simulink model "S_Med_TE_MPPT_Simp_V1"  (R2017a)
settings: Solver=FixedStepDiscrete  StartTime=0.0  StopTime=10.0  RelTol=1e-3
values from neighbouring files (symbols this model uses):
  A = [0 (d-1)/L ... (first row only)    [M_Mod_Sim_PV_V1.m]
  dIL = (vpv/L)*d*Ts1    (= 0.460350492963)    [M_Mod_Sim_PV_V1.m]
  Kf1 = Scala/dDmax    (= 5.88235294118)    [M_Mod_Sim_PV_V1.m]
  ki = 1/ipv    (= 0.0636345580933)    [M_Mod_Sim_PV_V1.m]
  Ts_Ma = 10e-3    (= 0.01)    [M_Mod_Sim_PV_V1.m]
undefined symbols (not defined in the file or in its folder): Down, GPTRIP1SEL, GPTRIP2SEL, TZ1, TZ2, Up
libraries: c2802xlib x4, c2806xlib x2, fuzblock x1
settings Model: ExtModeTrigDuration=8  Creator=dricl  LastModifiedBy=dricl
settings OptimizationCC: DefaultUnderspecifiedDataType=single  PassReuseOutputArgsAs=Individual arguments  MaxStackSize=512
settings DebuggingCC: ParameterTunabilityLossMsg=error
settings HardwareCC: ProdBitPerChar=16  ProdBitPerInt=16  ProdBitPerPointer=32  ProdBitPerSizeT=32  ProdBitPerPtrDiffT=32  ProdLargestAtomicInteger=Integer  ProdLargestAtomicFloat=None  ProdWordSize=16  ProdLongLongMode=on  ProdHWDeviceType=Texas Instruments->C2000
settings SFSimCC: MATLABDynamicMemAlloc=off
settings RTWCC: SystemTargetFile=ert.tlc  HardwareBoard=TI Piccolo F2806x  TLCOptions=-aInlineSetEventsForThisBaseRateFcn=TLC_FALSE -aSuppressMultiTaskScheduler=TLC_FALSE -aRateBasedStepFcn=1  TemplateMakefile=ert_default_tmf  Description=Embedded Coder  Toolchain=Texas Instruments Code Composer Studio v5 (C2000)  CodeExecutionProfiling=on  CodeProfilingSaveOptions=AllData  CodeProfilingInstrumentation=on
settings CodeAppCC: ForceParamTrailComments=on  IgnoreCustomStorageClasses=off  OperatorAnnotations=on  SimulinkDataObjDesc=on  SFDataObjDesc=on  MATLABFcnDesc=on  InsertBlockDesc=on  MATLABSourceComments=on
settings ERTTargetCC: CodeReplacementLibrary=TI C28x  MemSecPackage=tic2000demospkg  MemSecFuncExecute=code_ramfuncs

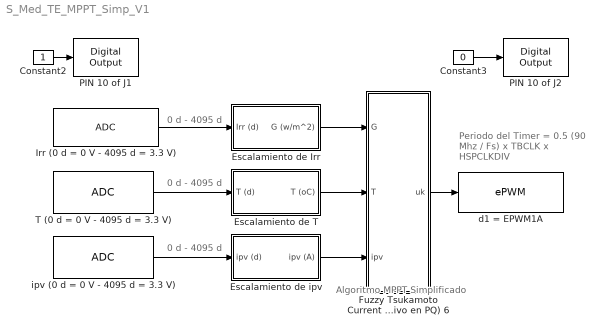
== system S_Med_TE_MPPT_Simp_V1 ==
  note: 0 d - 4095 d
  note: Periodo del Timer =
      |  0.5 (90 Mhz / Fs)  x
      | TBCLK x HSPCLKDIV
  note: 0 d - 4095 d
  note: 0 d - 4095 d
  note: Algoritmo MPPT Simplificado
  Constant2 : Constant  Priority=1  SampleTime=Ts_Ma
  Constant3 : Constant  Priority=11  Value=0  SampleTime=Ts_Ma
  Escalamiento de Irr : Subsystem  Priority=6  TreatAsAtomicUnit=on
  Escalamiento de T : Subsystem  Priority=7  TreatAsAtomicUnit=on
  Escalamiento de ipv : Subsystem  Priority=8  TreatAsAtomicUnit=on
  "Fuzzy Tsukamoto Current Controller n_mppt = 99.11%, ta(2%) = 0.12 s con Steps de Irrad Interv. 2 Seg. n_mppt = 96.74%, ta(2%) = 0.12 s con Steps de Irrad Interv. 0.5 Seg. n_mppt = 99.37%, ta(2%) = 0.12 s con Curva de Irrad Este controlador puede disminuir ta e incrementar a tr para mitigar los MP en id (impacto positivo en PQ) 6" : Subsystem  Priority=9
  "Irr (0 d = 0 V - 4095 d = 3.3 V) " : c2802xlib/ADC  Priority=3  ADCModule=1  samplingMode=Single sample mode  ADCResolution=12-bit (Single-ended input)  useSOC1=SOC1  useSOC2=SOC0_SOC1  SOCAcquisitionWindow=7  SOCTriggerSource=ePWM1_ADCSOCA  SOCInterruptTrigger=No ADCINT  Ts=Ts_Ma  dType=uint16  postInterrupt=off  interruptSel=ADCINT1  ADCINTContinuous=on  endma=off  chdma=1  blkParamProc=C2000  conv1=ADCINA1  conv2=ADCINA0 and ADCINB0  conv1_Type4=ADCIN0  conv2_Type4=ADCIN0 and ADCIN1
      settings: SourceProductName=Embedded Coder Support Package for Texas Instruments C2000 Processors
  PIN 10 of J1 : c2806xlib/Digital Output  Priority=2  GPIO_Number=GPIO32~GPIO39  GPIO_Bit0=on  GPIO_BIT0_Toggle=off  GPIO_Bit1=off  GPIO_BIT1_Toggle=off  GPIO_Bit2=off  GPIO_BIT2_Toggle=off  GPIO_Bit3=off  GPIO_BIT3_Toggle=off  GPIO_Bit4=off  GPIO_BIT4_Toggle=off  GPIO_Bit5=off  GPIO_BIT5_Toggle=off  GPIO_Bit6=off  GPIO_BIT6_Toggle=off  GPIO_Bit7=off  GPIO_BIT7_Toggle=off
      settings: SourceProductName=Embedded Coder Support Package for Texas Instruments C2000 Processors  SourceProductBaseCode=TIC2000
  PIN 10 of J2 : c2806xlib/Digital Output  Priority=12  GPIO_Number=GPIO32~GPIO39  GPIO_Bit0=on  GPIO_BIT0_Toggle=off  GPIO_Bit1=off  GPIO_BIT1_Toggle=off  GPIO_Bit2=off  GPIO_BIT2_Toggle=off  GPIO_Bit3=off  GPIO_BIT3_Toggle=off  GPIO_Bit4=off  GPIO_BIT4_Toggle=off  GPIO_Bit5=off  GPIO_BIT5_Toggle=off  GPIO_Bit6=off  GPIO_BIT6_Toggle=off  GPIO_Bit7=off  GPIO_BIT7_Toggle=off
      settings: SourceProductName=Embedded Coder Support Package for Texas Instruments C2000 Processors  SourceProductBaseCode=TIC2000
  "T (0 d = 0 V - 4095 d = 3.3 V) " : c2802xlib/ADC  Priority=4  ADCModule=1  samplingMode=Single sample mode  ADCResolution=12-bit (Single-ended input)  useSOC1=SOC3  useSOC2=SOC0_SOC1  SOCAcquisitionWindow=7  SOCTriggerSource=ePWM1_ADCSOCA  SOCInterruptTrigger=No ADCINT  Ts=Ts_Ma  dType=uint16  postInterrupt=off  interruptSel=ADCINT1  ADCINTContinuous=on  endma=off  chdma=1  blkParamProc=C2000  conv1=ADCINA2  conv2=ADCINA0 and ADCINB0  conv1_Type4=ADCIN0  conv2_Type4=ADCIN0 and ADCIN1
      settings: SourceProductName=Embedded Coder Support Package for Texas Instruments C2000 Processors
  d1 = EPWM1A : c2802xlib/ePWM  Priority=10  useModule=ePWM1  ePWMxLINKTBPRD=Not Linked  periodUnits=Clock cycles  timerSource=Specify via dialog  timerPeriod_clk=9000  timerPeriod_sec=0.0001  tbshadow=Counter equals to zero  countingMode=Up-Down  phaseActiveEnable=Disable  phaseDirection=Count down after sync  phaseActive=0  synchronizationEnable=off  dcaevt1Sync=off  dcbevt1Sync=off  synchronizationOption=Disable  clockPrescale=1  HSclockPrescale=1  enswap=off  ePWMxAStatus=on  ePWMxAactionLogic1=Do nothing  ePWMxAactionLogic2=Do nothing  ePWMxAactionLogic3=Clear  ePWMxAactionLogic4=Set  ePWMxAactionLogic5=Do nothing  ePWMxAactionLogic6=Do nothing  ePWMxALoadMode=Load on counter equals to zero (CTR=Zero)  ePWMxACSFenable=off  ePWMxACSFvalue=Forcing disable  ePWMxASFreload=Zero  ePWMxBStatus=off  ePWMxBactionLogic1=Set  ePWMxBactionLogic2=Clear  ePWMxBactionLogic3=Do nothing  ePWMxBactionLogic4=Do nothing  ePWMxBactionLogic5=Clear  ePWMxBactionLogic6=Set  ePWMxBLoadMode=Load on counter equals to zero (CTR=Zero)  ePWMxBCSFenable=off  ePWMxBCSFvalue=Forcing disable  ePWMxBSFreload=Zero  ePWNxBOutWay=off  ePWMxLINKCMPA=Not Linked  CMPAUnits=Clock cycles  CMPASource=Input port  CMPAValue_per=50  CMPAValue_clk=4500  enCMPAshadow=Counter equals to zero  ePWMxLINKCMPB=Not Linked  CMPBUnits=Clock cycles  CMPBSource=Specify via dialog  CMPBValue_per=50  CMPBValue_clk=4500  enCMPBshadow=Counter equals to zero  ePWMxLINKCMPC=Not Linked  CMPCUnits=Clock cycles  CMPCSource=Specify via dialog  CMPCValue_per=50  CMPCValue_clk=32000  enCMPCshadow=Counter equals to zero  ePWMxLINKCMPD=Not Linked  CMPDUnits=Clock cycles  CMPDSource=Specify via dialog  CMPDValue_per=50  CMPDValue_clk=32000  enCMPDshadow=Counter equals to zero  enableDBePWMxA=on  enableDBePWMxB=on  enhalfcycle=off  DBpolarity=Active high complementary (AHC)  DBedgeDelay=Positive  DBSource_ePWMxA=ePWMxA  DBSource_ePWMxB=ePWMxA  DBperiodSource=Specify via dialog  REDperiod=50  FEDperiod=50  adcstartModuleA=on  adcrequestEventA=First event  adcstartEventA=Counter equals to period (CTR=PRD)  adcstartEventA_type2=Digital Compare Module A Event 1 start of conversion (DCAEVT1.soc)  adcstartModuleB=off  adcrequestEventB=First event  adcstartEventB=Counter equals to zero (CTR=Zero)  adcstartEventB_type2=Counter equals to zero (CTR=Zero)  intEn=off  intPrd=First event  intSel=Counter equals to zero (CTR=Zero)  intSel_type2=Counter equals to zero (CTR=Zero)  hrpe=off  enHRPWM=off  HRPWM_LoadMode=Counter equals to period (CTR=PRD)  HRPWM_CTLMode=Duty or Period control mode  HRPWM_EDGMode=Both edge  hrpeb=off  enHRPWMB=off  HRPWM_LoadModeB=Counter equals to zero (CTR=ZERO)  HRPWM_CTLModeB=Duty or Period control mode  HRPWM_EDGModeB=Both edge  enSFO=on  enautoconv=on  chopperEnable=off  chopperFrequency=1  chopperFirstwidth=1  chopperDuty=12.5%  tripZonesource=Specify via dialog  tzselOSHT1=off  tzselOSHT2=off  tzselOSHT3=off  tzselOSHDCAEV1=off  tzselOSHDCBEV1=off  tzselCBC1=off  tzselCBC2=off  tzselCBC3=off  tzselCBCDCAEV2=off  tzselCBCDCBEV2=off  tzselOSHT4=off  tzselOSHT5=off  tzselOSHT6=off  tzselCBC4=off  tzselCBC5=off  tzselCBC6=off  enTzOstIntr=off  enTzCbcIntr=off  enTzDCAEVT1Intr=off  enTzDCAEVT2Intr=off  enTzDCBEVT1Intr=off  enTzDCBEVT2Intr=off  ePWMxAforced=No action  ePWMxBforced=No action  DCAEVT1forced=No action  DCBEVT1forced=No action  DCAEVT2forced=No action  DCBEVT2forced=No action  dcah=Trip Zone 1 input (TZ1)  dcal=Trip Zone 2 input (TZ2)  dcbh=Trip Zone 1 input (TZ1)  dcbl=Trip Zone 2 input (TZ2)  dcah_type2=GPTRIP1SEL/(TZ1)  dcal_type2=GPTRIP2SEL/(TZ2)  dcbh_type2=GPTRIP1SEL/(TZ1)  dcbl_type2=GPTRIP2SEL/(TZ2)  gendcaevt1=Event disabled  gendcaevt2=Event disabled  gendcbevt1=Event disabled  gendcbevt2=Event disabled  dcaevt1src=DCAEVT1 with sync  dcaevt2src=DCAEVT2 with sync  dcbevt1src=DCBEVT1 with sync  dcbevt2src=DCBEVT2 with sync  pulsesel=Counter equals to zero (CTR=Zero)  blankinv=off  blankoffset=0  blankwidth=0  evsrcsel=Filtered version of DCAEVT1 (DCAEVT1FILT)  encape=off  PwmType=C2000
      settings: SourceProductName=Embedded Coder Support Package for Texas Instruments C2000 Processors
  "ipv (0 d = 0 V - 4095 d = 3.3 V) " : c2802xlib/ADC  Priority=5  ADCModule=1  samplingMode=Single sample mode  ADCResolution=12-bit (Single-ended input)  useSOC1=SOC2  useSOC2=SOC0_SOC1  SOCAcquisitionWindow=7  SOCTriggerSource=ePWM1_ADCSOCA  SOCInterruptTrigger=No ADCINT  Ts=Ts_Ma  dType=uint16  postInterrupt=off  interruptSel=ADCINT1  ADCINTContinuous=on  endma=off  chdma=1  blkParamProc=C2000  conv1=ADCINA0  conv2=ADCINA0 and ADCINB0  conv1_Type4=ADCIN0  conv2_Type4=ADCIN0 and ADCIN1
      settings: SourceProductName=Embedded Coder Support Package for Texas Instruments C2000 Processors
  wires:
  "ipv (0 d = 0 V - 4095 d = 3.3 V) "/1 -> Escalamiento de ipv/1(ipv (d))
  "Irr (0 d = 0 V - 4095 d = 3.3 V) "/1 -> Escalamiento de Irr/1(Irr (d))
  Constant2/1 -> PIN 10 of J1/1
  Constant3/1 -> PIN 10 of J2/1
  "T (0 d = 0 V - 4095 d = 3.3 V) "/1 -> Escalamiento de T/1(T (d))
  Escalamiento de Irr/1(G (w/m^2)) -> "Fuzzy Tsukamoto Current Controller n_mppt = 99.11%, ta(2%) = 0.12 s con Steps de Irrad Interv. 2 Seg. n_mppt = 96.74%, ta(2%) = 0.12 s con Steps de Irrad Interv. 0.5 Seg. n_mppt = 99.37%, ta(2%) = 0.12 s con Curva de Irrad Este controlador puede disminuir ta e incrementar a tr para mitigar los MP en id (impacto positivo en PQ) 6"/1(G)
  Escalamiento de T/1(T (oC)) -> "Fuzzy Tsukamoto Current Controller n_mppt = 99.11%, ta(2%) = 0.12 s con Steps de Irrad Interv. 2 Seg. n_mppt = 96.74%, ta(2%) = 0.12 s con Steps de Irrad Interv. 0.5 Seg. n_mppt = 99.37%, ta(2%) = 0.12 s con Curva de Irrad Este controlador puede disminuir ta e incrementar a tr para mitigar los MP en id (impacto positivo en PQ) 6"/2(T)
  Escalamiento de ipv/1(ipv (A)) -> "Fuzzy Tsukamoto Current Controller n_mppt = 99.11%, ta(2%) = 0.12 s con Steps de Irrad Interv. 2 Seg. n_mppt = 96.74%, ta(2%) = 0.12 s con Steps de Irrad Interv. 0.5 Seg. n_mppt = 99.37%, ta(2%) = 0.12 s con Curva de Irrad Este controlador puede disminuir ta e incrementar a tr para mitigar los MP en id (impacto positivo en PQ) 6"/3(ipv)
  "Fuzzy Tsukamoto Current Controller n_mppt = 99.11%, ta(2%) = 0.12 s con Steps de Irrad Interv. 2 Seg. n_mppt = 96.74%, ta(2%) = 0.12 s con Steps de Irrad Interv. 0.5 Seg. n_mppt = 99.37%, ta(2%) = 0.12 s con Curva de Irrad Este controlador puede disminuir ta e incrementar a tr para mitigar los MP en id (impacto positivo en PQ) 6"/1(uk) -> d1 = EPWM1A/1

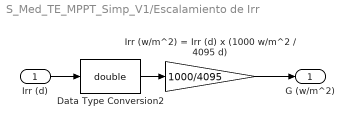
== system S_Med_TE_MPPT_Simp_V1/Escalamiento de Irr ==
  Irr (d) : Inport
  Data Type Conversion2 : DataTypeConversion  OutDataTypeStr=double
  Irr (w/m^2) = Irr (d) x (1000 w/m^2 / 4095 d) : Gain  Gain=1000/4095
  G (w/m^2) : Outport
  wires:
  Irr (d)/1 -> Data Type Conversion2/1
  Data Type Conversion2/1 -> Irr (w/m^2) = Irr (d) x (1000 w/m^2 / 4095 d)/1
  Irr (w/m^2) = Irr (d) x (1000 w/m^2 / 4095 d)/1 -> G (w/m^2)/1

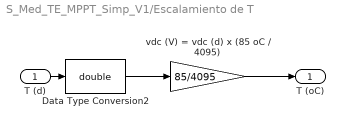
== system S_Med_TE_MPPT_Simp_V1/Escalamiento de T ==
  T (d) : Inport
  Data Type Conversion2 : DataTypeConversion  OutDataTypeStr=double
  vdc (V) = vdc (d) x (85 oC / 4095) : Gain  Gain=85/4095
  T (oC) : Outport
  wires:
  Data Type Conversion2/1 -> vdc (V) = vdc (d) x (85 oC / 4095)/1
  T (d)/1 -> Data Type Conversion2/1
  vdc (V) = vdc (d) x (85 oC / 4095)/1 -> T (oC)/1

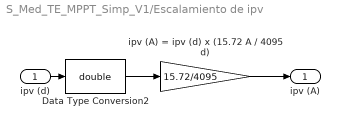
== system S_Med_TE_MPPT_Simp_V1/Escalamiento de ipv ==
  ipv (d) : Inport
  Data Type Conversion2 : DataTypeConversion  OutDataTypeStr=double
  ipv (A) = ipv (d) x (15.72 A / 4095 d) : Gain  Gain=15.72/4095
  ipv (A) : Outport
  wires:
  ipv (d)/1 -> Data Type Conversion2/1
  Data Type Conversion2/1 -> ipv (A) = ipv (d) x (15.72 A / 4095 d)/1
  ipv (A) = ipv (d) x (15.72 A / 4095 d)/1 -> ipv (A)/1

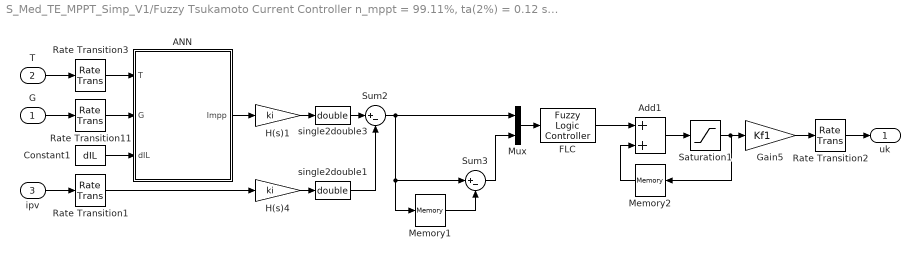
== system S_Med_TE_MPPT_Simp_V1/Fuzzy Tsukamoto Current Controller n_mppt = 99.11%, ta(2%) = 0.12 s con Steps de Irrad Interv. 2 Seg. n_mppt = 96.74%, ta(2%) = 0.12 s con Steps de Irrad Interv. 0.5 Seg. n_mppt = 99.37%, ta(2%) = 0.12 s con Curva de Irrad Este controlador puede disminuir ta e incrementar a tr para mitigar los MP en id (impacto positivo en PQ) 6 ==
  G : Inport
  T : Inport  Port=2
  ipv : Inport  Port=3
  ANN : MATLAB Function  TreatAsAtomicUnit=on
  Add1 : Sum
  Constant1 : Constant  Value=dIL  SampleTime=Ts_Ma
  FLC : fuzblock/Fuzzy Logic  Controller  fis=['5_Rules_MaMPPTCtrl_V1.fis']
  Gain5 : Gain  Gain=Kf1
  H(s)1 : Gain  Gain=ki
  H(s)4 : Gain  Gain=ki
  Memory1 : Memory  InheritSampleTime=on
  Memory2 : Memory  InheritSampleTime=on
  Mux : Mux  Inputs=2
  Rate Transition{1..3,11} (4 alike) : RateTransition  Deterministic=off  OutPortSampleTime=Ts_Ma
  Saturation1 : Saturate  UpperLimit=1  LowerLimit=0
  Sum2 : Sum  Inputs=|+-
  Sum3 : Sum  Inputs=|+-
  single2double1 : DataTypeConversion  OutDataTypeStr=double
  single2double3 : DataTypeConversion  OutDataTypeStr=double
  uk : Outport
  wires:
  Rate Transition2/1 -> uk/1
  Memory2/1 -> Add1/2
  single2double3/1 -> Sum2/1
  single2double1/1 -> Sum2/2
  Rate Transition1/1 -> H(s)4/1
  ipv/1 -> Rate Transition1/1
  Memory1/1 -> Sum3/2
  Add1/1 -> Saturation1/1
  Saturation1/1 -> Memory2/1, Gain5/1
  Gain5/1 -> Rate Transition2/1
  H(s)1/1 -> single2double3/1
  H(s)4/1 -> single2double1/1
  Mux/1 -> FLC/1
  Sum2/1 -> Memory1/1, Sum3/1, Mux/1
  Sum3/1 -> Mux/2
  FLC/1 -> Add1/1
  Rate Transition11/1 -> ANN/2(G)
  Rate Transition3/1 -> ANN/1(T)
  G/1 -> Rate Transition11/1
  T/1 -> Rate Transition3/1
  Constant1/1 -> ANN/3(dIL)
  ANN/1(Impp) -> H(s)1/1

== matlab function S_Med_TE_MPPT_Simp_V1/Fuzzy Tsukamoto Current Controller n_mppt = 99.11%, ta(2%) = 0.12 s con Steps de Irrad Interv. 2 Seg. n_mppt = 96.74%, ta(2%) = 0.12 s con Steps de Irrad Interv. 0.5 Seg. n_mppt = 99.37%, ta(2%) = 0.12 s con Curva de Irrad Este controlador puede disminuir ta e incrementar a tr para mitigar los MP en id (impacto positivo en PQ) 6/ANN ==
  data: T input; G input; Impp output; dIL input
function Impp = ANN(T,G,dIL)

persistent w1 w2 b1 b2
persistent Media_T Media_G Media_Impp
persistent Std_T Std_G Std_Impp

if isempty(w1)

    w1 = [ ...
    0.0800025921861489, -0.2701751801560736; ...
    0.0593520039763442, -0.2027427120547354; ...
    0.5243220553759315, 0.1630350434999212; ...
    1.5863696961889453, 0.1819964305283979; ...
    -6.2441844424671862, -2.3703350404983592];

    w2 = [-8.8999407900435337, -14.3986509522404820, 2.0426767954493643, 0.2264966677997083, -0.0152565567604669];

    b1 = [-1.5663442358887940, 0.9898870290888165, -0.3688041794616991, 2.4837588514086595, -13.7136306663382130];

    b2 = 10.9993641444783350;

    Media_T = 30.0000000000000000;
    Media_G = 650.0000000000000000;
    Media_Impp = 10.2067479487858090;

    Std_T = 32.3328756401525790;
    Std_G = 324.7437686605284200;
    Std_Impp = 5.0831144693742818;
    
end

%% =========================================================
% NORMALIZACION
% ==========================================================
% La red fue entrenada con:
%   x1 = T normalizada
%   x2 = G normalizada
%
% Por eso, antes de evaluar la ANN se aplica la misma
% normalización usada durante el entrenamiento.

x1 = (T - Media_T)/Std_T;
x2 = (G - Media_G)/Std_G;

%% =========================================================
% CAPA OCULTA
% ==========================================================
% Cada neurona oculta usa función logsig:
%
%   logsig(n) = 1/(1+exp(-n))

N1 = b1(1) + x1*w1(1,1) + x2*w1(1,2);
N1 = 1/(1+exp(-N1));

N2 = b1(2) + x1*w1(2,1) + x2*w1(2,2);
N2 = 1/(1+exp(-N2));

N3 = b1(3) + x1*w1(3,1) + x2*w1(3,2);
N3 = 1/(1+exp(-N3));

N4 = b1(4) + x1*w1(4,1) + x2*w1(4,2);
N4 = 1/(1+exp(-N4));

N5 = b1(5) + x1*w1(5,1) + x2*w1(5,2);
N5 = 1/(1+exp(-N5));

%% =========================================================
% CAPA DE SALIDA
% ==========================================================
% La salida de la red está normalizada.

Salida_norm = b2 + ...
              N1*w2(1,1) + ...
              N2*w2(1,2) + ...
              N3*w2(1,3) + ...
              N4*w2(1,4) + ...
              N5*w2(1,5);

%% =========================================================
% DESNORMALIZACION
% ==========================================================
% Se convierte la salida normalizada a amperes.

Impp_nom = Salida_norm*Std_Impp + Media_Impp;

%% =========================================================
% CORRECCION POR RIZO DE CORRIENTE dIL
% ==========================================================
% La ANN entrega una referencia nominal Impp_nom.
%
% dIL representa el rizo pico-a-pico de la corriente del inductor.
% Al restar dIL, la referencia se desplaza hacia abajo para evitar
% que la envolvente superior del rizo supere la corriente Impp.
%
% Esto es equivalente a:
%
%   Iref = Impp_nom - dIL
%
% Finalmente se satura a cero para evitar referencias negativas.

Impp = Impp_nom - dIL;

% Saturación inferior
Impp = max(Impp,0);

end
